simulink model "capacitor_voltripple"  (R2013a)
settings: Solver=ode4  StartTime=0.0  StopTime=0.12  FixedStep=Ts  RelTol=1e-3
values from neighbouring files (symbols this model uses):
  Cdc = 50e-6    (= 5e-05)    [immd_capacitor_rms_current.m]    (also in immd_design_elen.m = 0.0002; immd_efficiency.m; immd_simulation_base.m; sixth_harmonic_report.m = 0.003)
  Lload = Xload/wout_fund    [acemp_sixth.m]    (also in immd_base_varyingmod.m = Xload/wout; immd_design_elen.m = Xload/wout; immd_efficiency.m = Xload/wout; immd_simulation_base.m = Xload/wout)
  ma = 1    [IMMD_design_tool_v01.m]    (also in IMMD_design_tool_v02.m = 0.9; immd_base_varyingmod.m; immd_design_elen.m = 0.8; immd_efficiency.m = 0.85)
  R1 = 5    [immd_efficiency.m]    (also in immd_simulation_base.m)
  Rload = Zload*pf    [acemp_sixth.m]    (also in immd_base_varyingmod.m; immd_design_elen.m; immd_efficiency.m; immd_simulation_base.m)
  Ts = 1e-6    (= 1e-06)    [acemp_sixth.m]    (also in immd_base_varyingmod.m = 1e-05; immd_design_elen.m; immd_efficiency.m; immd_simulation_base.m)
  V1 = Vdc*(R1+Rrefl)/Rrefl    (= 526.262626263)    [immd_efficiency.m]    (also in immd_simulation_base.m = 425.252525253)
  wout = 2*pi*fout    (= 314.159265359)    [immd_base_varyingmod.m]    (also in immd_design_elen.m; immd_efficiency.m; immd_simulation_base.m)
libraries: powerlib x23, powerlib_meascontrol x8, simulink x2
settings Model: Creator=ugurm  LastModifiedBy=ugurm

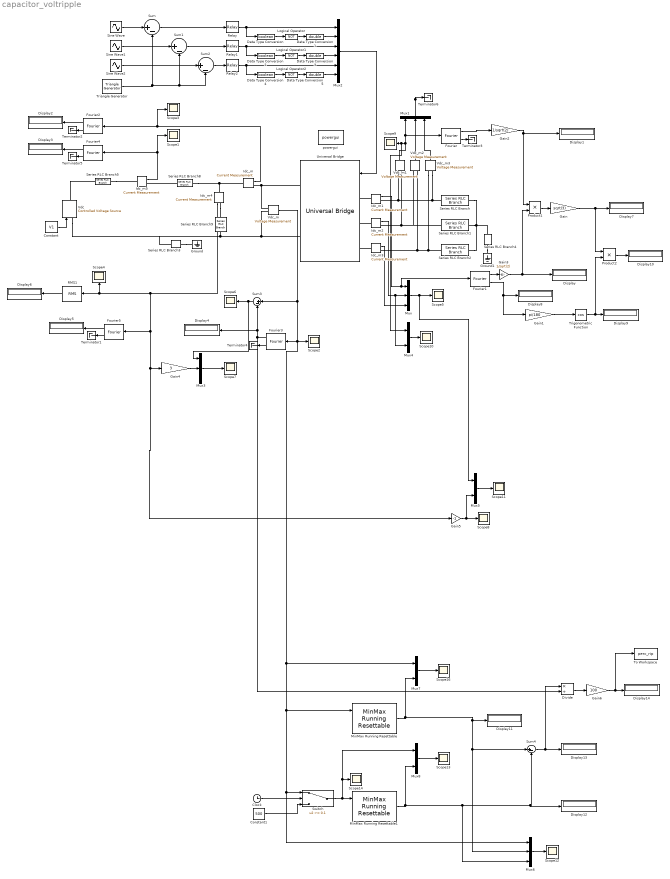
== system capacitor_voltripple ==
  Clock : Clock
  Constant : Constant  Value=V1
  Constant1 : Constant  Value=500  SampleTime=Ts
  Data Type Conversion : DataTypeConversion  OutDataTypeStr=boolean
  Data Type Conversion1 : DataTypeConversion  OutDataTypeStr=double
  Data Type Conversion2 : DataTypeConversion  OutDataTypeStr=boolean
  Data Type Conversion3 : DataTypeConversion  OutDataTypeStr=double
  Data Type Conversion4 : DataTypeConversion  OutDataTypeStr=boolean
  Data Type Conversion5 : DataTypeConversion  OutDataTypeStr=double
  Display{,1..14} (15 alike) : Display
      Display7 settings: Format=short_e
  Divide : Product  Inputs=*/
  Fourier : powerlib_meascontrol/Measurements/Fourier  Freq=fout  n=1  InInit=[0, 0]  Ts=Ts
  Fourier1 : powerlib_meascontrol/Measurements/Fourier  Freq=fout  n=1  InInit=[0, 0]  Ts=Ts
  Fourier{2..5} (4 alike) : powerlib_meascontrol/Measurements/Fourier  Freq=fout  n=0  InInit=[0, 0]  Ts=Ts
  Gain : Gain  Gain=sqrt(3)
  Gain1 : Gain  Gain=pi/180
  Gain2 : Gain  Gain=1/sqrt(2)
  Gain3 : Gain  Gain=1/sqrt(2)
  Gain4 : Gain  Gain=3
  Gain5 : Gain  Gain=-1
  Gain6 : Gain  Gain=100
  Ground : powerlib/Elements/Ground  LConnTagsString=a
  Ground1 : powerlib/Elements/Ground  LConnTagsString=a
  Idc_m{,1..5} (6 alike) : powerlib/Measurements/Current Measurement  PhasorSimulation=off  OutputType=Complex  PSBequivalent=0
  Logical Operator : Logic  Operator=NOT  AllPortsSameDT=off  OutDataTypeStr=boolean
  Logical Operator1 : Logic  Operator=NOT  AllPortsSameDT=off  OutDataTypeStr=boolean
  Logical Operator2 : Logic  Operator=NOT  AllPortsSameDT=off  OutDataTypeStr=boolean
  MinMax Running Resettable : simulink/Math Operations/MinMax Running Resettable  Function=max  vinit=0.0
  MinMax Running Resettable1 : simulink/Math Operations/MinMax Running Resettable  Function=min  vinit=500
  Mux{,1,3,6} (4 alike) : Mux  Inputs=3
  Mux2 : Mux  Inputs=6
  Mux{4..5,7..8} (4 alike) : Mux  Inputs=2
  Product1 : Product
  Product2 : Product
  RMS1 : powerlib_meascontrol/Measurements/RMS  TrueRMS=on  Freq=50  RMSInit=120  Ts=Ts
  Relay : Relay
  Relay1 : Relay
  Relay2 : Relay
  Scope{1..14,16} (15 alike) : Scope
      Scope1 settings: YMin=3.6  YMax=5.1
      Scope10 settings: YMin=-450  YMax=450  SaveName=ScopeData9
      Scope11 settings: YMin=-5.5  YMax=3  SaveName=ScopeData10
      Scope12 settings: YMin=385  YMax=500  SaveName=ScopeData11
      Scope13 settings: YMin=385  YMax=500  SaveName=ScopeData12
      Scope14 settings: YMin=500  YMax=500  SaveName=ScopeData13
      Scope16 settings: YMin=367.5  YMax=415  SaveName=ScopeData15
      Scope2 settings: YMin=150  YMax=550  SaveName=ScopeData2
      Scope3 settings: YMin=500  YMax=800  SaveName=ScopeData3
      Scope4 settings: YMin=500  YMax=800  SaveName=ScopeData4
      Scope5 settings: YMin=500  YMax=800
      Scope6 settings: YMin=475  YMax=975  SaveName=ScopeData5
      Scope7 settings: YMin=-25  YMax=350  SaveName=ScopeData6
      Scope8 settings: YMin=-5.5  YMax=3  SaveName=ScopeData7
      Scope9 settings: YMin=-450  YMax=450  SaveName=ScopeData8
  Series RLC Branch : powerlib/Elements/Series RLC Branch  LConnTagsString=__new0  RConnTagsString=__new0  BranchType=RL  Resistance=Rload  Inductance=Lload  SetiL0=off  InitialCurrent=0  Capacitance=1e-6  Setx0=off  InitialVoltage=0  Measurements=None
  Series RLC Branch1 : powerlib/Elements/Series RLC Branch  LConnTagsString=__new0  RConnTagsString=__new0  BranchType=RL  Resistance=Rload  Inductance=Lload  SetiL0=off  InitialCurrent=0  Capacitance=1e-6  Setx0=off  InitialVoltage=0  Measurements=None
  Series RLC Branch2 : powerlib/Elements/Series RLC Branch  LConnTagsString=__new0  RConnTagsString=__new0  BranchType=RL  Resistance=Rload  Inductance=Lload  SetiL0=off  InitialCurrent=0  Capacitance=1e-6  Setx0=off  InitialVoltage=0  Measurements=None
  Series RLC Branch3 : powerlib/Elements/Series RLC Branch  LConnTagsString=__new0  RConnTagsString=__new0  BranchType=R  Resistance=1e12  Inductance=Lload  SetiL0=off  InitialCurrent=0  Capacitance=1e-6  Setx0=off  InitialVoltage=0  Measurements=None
  Series RLC Branch4 : powerlib/Elements/Series RLC Branch  LConnTagsString=__new0  RConnTagsString=__new0  BranchType=R  Resistance=1e12  Inductance=Lload  SetiL0=off  InitialCurrent=0  Capacitance=1e-6  Setx0=off  InitialVoltage=0  Measurements=None
  Series RLC Branch5 : powerlib/Elements/Series RLC Branch  LConnTagsString=__new0  RConnTagsString=__new0  BranchType=L  Resistance=1  Inductance=1  SetiL0=off  InitialCurrent=0  Capacitance=1e-6  Setx0=off  InitialVoltage=0  Measurements=None
  Series RLC Branch8 : powerlib/Elements/Series RLC Branch  LConnTagsString=__new0  RConnTagsString=__new0  BranchType=R  Resistance=R1  Inductance=Lload  SetiL0=off  InitialCurrent=0  Capacitance=1e-6  Setx0=off  InitialVoltage=0  Measurements=None
  Series RLC Branch9 : powerlib/Elements/Series RLC Branch  LConnTagsString=__new0  RConnTagsString=__new0  BranchType=C  Resistance=1e12  Inductance=Lload  SetiL0=off  InitialCurrent=0  Capacitance=Cdc  Setx0=off  InitialVoltage=0  Measurements=None
  Sine Wave : Sin  Amplitude=ma  Frequency=wout  SampleTime=0
  Sine Wave1 : Sin  Amplitude=ma  Frequency=wout  Phase=-2*pi/3  SampleTime=0
  Sine Wave2 : Sin  Amplitude=ma  Frequency=wout  Phase=2*pi/3  SampleTime=0
  Sum{,1..4} (5 alike) : Sum  Inputs=|+-
  Switch : Switch  Threshold=0.1
  Terminator{1..6} (6 alike) : Terminator
  To Workspace : ToWorkspace  VariableName=perc_rip  SampleTime=Ts
  Triangle Generator : powerlib_meascontrol/Pulse & Signal Generators/Triangle Generator  Freq=fsw  Phase=0  Ts=Ts
  Trigonometric Function : Trigonometry  Operator=cos
  Universal Bridge : powerlib/Power Electronics/Universal Bridge  Arms=3  SnubberResistance=1e5  SnubberCapacitance=inf  Device=IGBT / Diodes  Ron=1e-6  Lon=0  ForwardVoltages="[  0  0  ]"  ForwardVoltage=0  GTOparameters=[ 10e-6 , 20e-6 ]  IGBTparameters=[ 1e-6 , 2e-6 ]  Measurements=None  Measurements_2=None  converterType=Rectifier
  Vdc : powerlib/Electrical Sources/Controlled Voltage Source  Initialize=off  Source_Type=DC  Amplitude=200  Phase=0  Frequency=0  Measurements=None
  Vdc_m{,1..3} (4 alike) : powerlib/Measurements/Voltage Measurement  PhasorSimulation=off  OutputType=Complex  PSBequivalent=0
  powergui : powerlib/powergui  Priority=1  SimulationMode=Discrete  SolverType=Tustin  SampleTime=Ts  frequency=60  SPID=off  DisableSnubberDevices=off  DisableRonSwitches=off  DisableVfSwitches=off  SwTol=0  Interpol=off  DisplayEquations=off  frequencyindice=0  Pbase=100e6  ErrMax=1e-4  Iterations=50  UnitsV=kV  UnitsW=MW  FunctionMessages=off  echomessages=off  HookPort=off  EnableUseOfTLC=off  x0status=blocks  RestoreLinks=warning  ResistiveCurrentMeasurement=off  Frange=[0:2:500]  Ylog=off  Xlog=on  ShowGrid=off  save=off  variable=ZData  structure=idc  ZoomFFT=off  StartTime=0.1  cycles=20  DisplayStyle=5  fundamental=50  FreqAxis=off  MaxFrequency=20000  frequencyindicesteady=1  RmsSteady=1  display=off  Ts=0  methode=off
  wires:
  Constant/1 -> Vdc/1
  Idc_m/1 -> Scope3/1, Fourier2/1
  Idc_m1/1 -> Fourier1/1, Mux/1
  Idc_m2/1 -> Mux4/2, Mux/2
  Idc_m3/1 -> Mux/3
  Mux/1 -> Mux5/1, Scope5/1
  Sine Wave/1 -> Sum/1
  Triangle Generator/1 -> Sum1/2, Sum2/2, Sum/2
  Sine Wave1/1 -> Sum1/1
  Sine Wave2/1 -> Sum2/1
  Sum/1 -> Relay/1
  Sum1/1 -> Relay1/1
  Sum2/1 -> Relay2/1
  Data Type Conversion/1 -> Logical Operator/1
  Relay/1 -> Data Type Conversion/1, Mux2/1
  Logical Operator/1 -> Data Type Conversion1/1
  Data Type Conversion1/1 -> Mux2/2
  Data Type Conversion2/1 -> Logical Operator1/1
  Relay1/1 -> Data Type Conversion2/1, Mux2/3
  Logical Operator1/1 -> Data Type Conversion3/1
  Data Type Conversion3/1 -> Mux2/4
  Data Type Conversion4/1 -> Logical Operator2/1
  Relay2/1 -> Data Type Conversion4/1, Mux2/5
  Logical Operator2/1 -> Data Type Conversion5/1
  Data Type Conversion5/1 -> Mux2/6
  Mux2/1 -> Universal Bridge/1
  Fourier1/1 -> Gain3/1
  Vdc_m1/1 -> Mux4/1, Scope9/1, Mux1/1, Fourier/1
  Vdc_m2/1 -> Mux1/2
  Vdc_m3/1 -> Mux1/3
  Fourier2/1 -> Display2/1
  Product1/1 -> Gain/1
  Gain/1 -> Product2/1, Display7/1
  Fourier1/2 -> Display8/1, Gain1/1
  Trigonometric Function/1 -> Product2/2, Display9/1
  Gain1/1 -> Trigonometric Function/1
  Product2/1 -> Display10/1
  Mux1/1 -> Terminator6/1
  Fourier2/2 -> Terminator2/1
  Fourier/2 -> Terminator3/1
  Fourier3/1 -> Sum3/2, Display4/1, Divide/2
  Fourier3/2 -> Terminator4/1
  Idc_m4/1 -> Fourier5/1, Gain5/1, Gain4/1, RMS1/1, Scope4/1
  RMS1/1 -> Display6/1
  Idc_m5/1 -> Scope1/1, Fourier4/1
  Fourier4/1 -> Display3/1
  Fourier4/2 -> Terminator5/1
  Gain2/1 -> Display1/1, Product1/1
  Fourier/1 -> Gain2/1
  Gain3/1 -> Display/1, Product1/2
  Fourier5/1 -> Display5/1
  Fourier5/2 -> Terminator1/1
  Sum3/1 -> Mux3/1, Scope6/1
  Mux3/1 -> Scope7/1
  Gain4/1 -> Mux3/2
  Gain5/1 -> Mux5/2, Scope8/1
  Mux4/1 -> Scope10/1
  Mux5/1 -> Scope11/1
  MinMax Running Resettable/1 -> Display11/1, Mux6/2, Sum4/1, Mux7/2
  Mux7/1 -> Scope16/1
  Vdc_m/1 -> Mux7/1, Mux6/1, Switch/1, MinMax Running Resettable/1, Fourier3/1, Scope2/1, Sum3/1
  MinMax Running Resettable1/1 -> Mux6/3, Display12/1, Sum4/2, Mux8/2
  Mux8/1 -> Scope13/1
  Switch/1 -> Mux8/1, Scope14/1, MinMax Running Resettable1/1
  Clock/1 -> Switch/2
  Constant1/1 -> Switch/3
  Sum4/1 -> Divide/1, Display13/1
  Divide/1 -> Gain6/1
  Gain6/1 -> To Workspace/1, Display14/1
  Mux6/1 -> Scope12/1
  connections:
  Universal Bridge/RConn1 -- Vdc_m/LConn1 -- Idc_m/RConn1
  Universal Bridge/RConn2 -- Vdc_m/LConn2 -- Vdc/LConn1 -- Series RLC Branch3/LConn1 -- Series RLC Branch9/RConn1
  Idc_m1/LConn1 -- Universal Bridge/LConn1
  Idc_m2/LConn1 -- Universal Bridge/LConn2
  Idc_m3/LConn1 -- Universal Bridge/LConn3
  Vdc_m3/LConn1 -- Series RLC Branch2/LConn1 -- Vdc_m2/LConn2 -- Idc_m3/RConn1
  Series RLC Branch1/LConn1 -- Vdc_m2/LConn1 -- Vdc_m1/LConn2 -- Idc_m2/RConn1
  Series RLC Branch/LConn1 -- Vdc_m3/LConn2 -- Vdc_m1/LConn1 -- Idc_m1/RConn1
  Series RLC Branch/RConn1 -- Series RLC Branch4/LConn1 -- Series RLC Branch2/RConn1 -- Series RLC Branch1/RConn1
  Series RLC Branch3/RConn1 -- Ground/LConn1
  Series RLC Branch4/RConn1 -- Ground1/LConn1
  Series RLC Branch8/LConn1 -- Idc_m4/LConn1 -- Idc_m/LConn1
  Idc_m4/RConn1 -- Series RLC Branch9/LConn1
  Series RLC Branch8/RConn1 -- Idc_m5/RConn1
  Series RLC Branch5/LConn1 -- Idc_m5/LConn1
  Series RLC Branch5/RConn1 -- Vdc/RConn1
